simulink model "part_iisim"  (R2021a)
settings: Solver=VariableStepAuto  StartTime=0.0  StopTime=30  RelTol=1e-6
undefined symbols (not defined in the file): cp, g, h, Jp_prime, m, th0
settings Model: Creator=Joseph  LastModifiedBy=Joseph

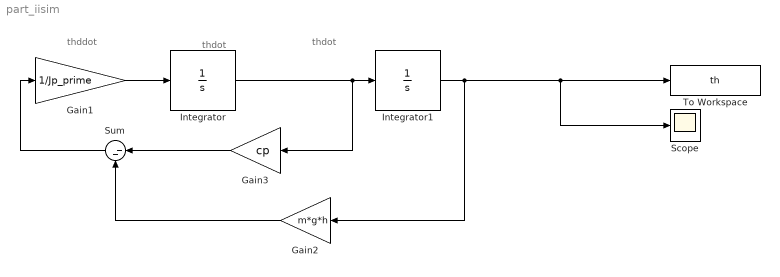
== system part_iisim ==
  note: thdot
  note: thddot
  note: thdot
  Gain1 : Gain  Gain=1/Jp_prime
  Gain2 : Gain  Gain=m*g*h
  Gain3 : Gain  Gain=cp
  Integrator : Integrator
  Integrator1 : Integrator  InitialCondition=th0
  Scope : Scope
  Sum : Sum  Inputs=|--
  To Workspace : ToWorkspace  VariableName=th  SaveFormat=Timeseries  SampleTime=-1
  wires:
  Integrator/1 -> Gain3/1, Integrator1/1
  Gain1/1 -> Integrator/1
  Integrator1/1 -> Scope/1, To Workspace/1, Gain2/1
  Gain2/1 -> Sum/2
  Sum/1 -> Gain1/1
  Gain3/1 -> Sum/1
